simulink model "bidireUnitfinal"  (R2024b)
settings: Solver=VariableStepAuto  StartTime=0.0  StopTime=10  RelTol=1e-3
model workspace (MAT data in the model file):
  charge = 1
undefined symbols (not defined in the file): Ion, Lithium
libraries: spsSeriesRLCBranchLib x3, spsBatteryLib x2, spsMosfetLib x2, spsVoltageMeasurementLib x2, spsCurrentMeasurementLib x1, slpidlib x1, spsTriangleGeneratorLib x1, spspowerguiLib x1
settings Model: Creator=pansi  LastModifiedBy=ASUS

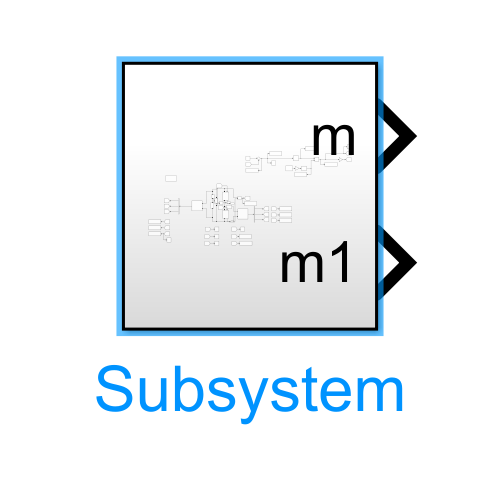
[thumbnail: Simulink's stored preview of the top-level diagram]
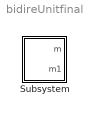
== system bidireUnitfinal ==
  Subsystem : Subsystem

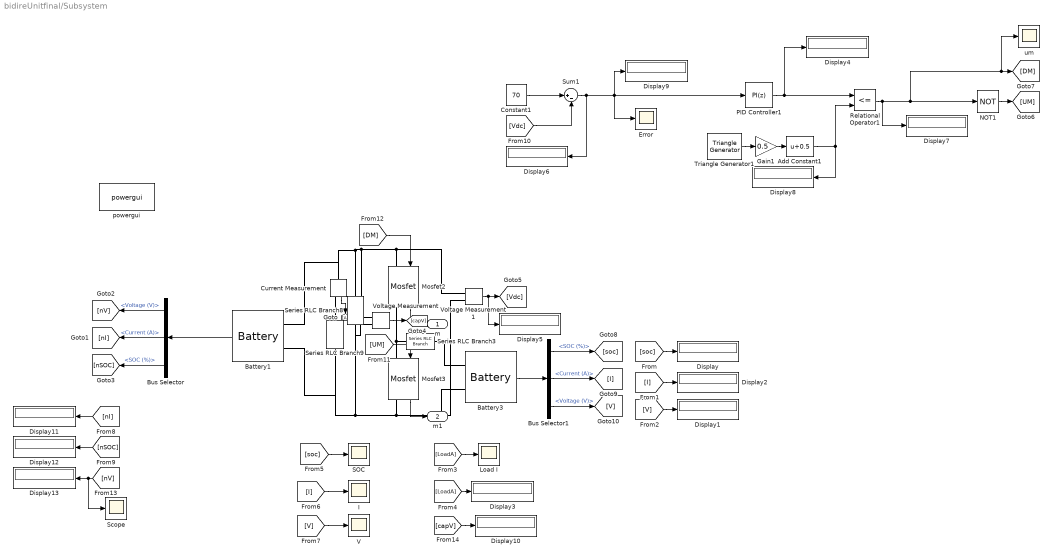
== system bidireUnitfinal/Subsystem ==
  Add Constant1 : Bias  Bias=0.5  SaturateOnIntegerOverflow=off
  Battery1 : spsBatteryLib/Battery  BatType=Lithium-Ion  NomV=25  NomQ=20  SOC=60  Batt_Tr=30  PresetModel=on  MaxQ=20  MinV=18.75  FullV=29.0997  Dis_rate=8.6957  R=0.0125  Normal_OP=18.087  expZone="[27.0096     0.982609]"
  Battery3 : spsBatteryLib/Battery  BatType=Lithium-Ion  NomV=50  NomQ=20  SOC=60  Batt_Tr=30  PresetModel=on  MaxQ=20  MinV=37.5  FullV=58.1994  Dis_rate=8.6957  R=0.025  Normal_OP=18.087  expZone="[54.0193     0.982609]"
  Bus Selector : BusSelector  OutputSignals=Voltage (V),Current (A),SOC (%)
  Bus Selector1 : BusSelector  OutputSignals=SOC (%),Current (A),Voltage (V)
  Constant1 : Constant  Value=70
  Current Measurement : spsCurrentMeasurementLib/Current Measurement  PhasorSimulation=off  OutputType=Complex  PSBequivalent=0
  Display{,1..13} (14 alike) : Display
  Error : Scope
  Gain1 : Gain  Gain=0.5
  Goto : Goto
  I : Scope
  Load I : Scope
  Mosfet2 : spsMosfetLib/Mosfet  Ron=0.1  Lon=0  Rd=0.01  Vfd=0  IC=0  Rs=1e6  Cs=inf  Measurements=on
  Mosfet3 : spsMosfetLib/Mosfet  Ron=0.1  Lon=0  Rd=0.01  Vfd=0  IC=0  Rs=1e6  Cs=inf  Measurements=on
  NOT1 : Logic  Operator=NOT  IconShape=distinctive  AllPortsSameDT=off  OutDataTypeStr=boolean
  PID Controller1 : slpidlib/PID Controller  Controller=PI  Form=Parallel  TimeDomain=Discrete-time  UseExternalTs=off  SampleTime=-1  IntegratorMethod=Forward Euler  FilterMethod=Forward Euler  ControllerParametersSource=internal  P=1  I=50  UseKiTs=off  D=0  UseExternalDerivativeSource=off  N=100  UseFilter=on  TunerSelectOption=Transfer Function Based (PID Tuner App)  ZeroCross=off  InitialConditionSource=internal  InitialConditionForIntegrator=0  InitialConditionForFilter=0  DifferentiatorICPrevScaledInput=0  ExternalReset=none  TrackingMode=off  Kt=1  LimitOutput=on  SatLimitsSource=internal  UpperSaturationLimit=1  LowerSaturationLimit=-1  LinearizeAsGain=on  AntiWindupMode=back-calculation  Kb=1  LimitIntegrator=off  UpperIntegratorSaturationLimit=inf  LowerIntegratorSaturationLimit=-inf  POutMin=[]  POutMax=[]  IOutMin=[]  IOutMax=[]  DOutMin=[]  DOutMax=[]  NOutMin=[]  NOutMax=[]  SumOutMin=[]  SumOutMax=[]  SaturationOutMin=[]  SaturationOutMax=[]  PParamMin=[]  PParamMax=[]  IParamMin=[]  IParamMax=[]  DParamMin=[]  DParamMax=[]  NParamMin=[]  NParamMax=[]  KbParamMin=[]  KbParamMax=[]  KtParamMin=[]  KtParamMax=[]  KbOutMin=[]  KbOutMax=[]  KtOutMin=[]  KtOutMax=[]  IntegratorOutMin=[]  IntegratorOutMax=[]  FilterOutMin=[]  FilterOutMax=[]  SumI1OutMin=[]  SumI1OutMax=[]  SumI2OutMin=[]  SumI2OutMax=[]  SumI3OutMin=[]  SumI3OutMax=[]  SumI4OutMin=[]  SumI4OutMax=[]  SumDOutMin=[]  SumDOutMax=[]  DifferentiatorOutMin=[]  DifferentiatorOutMax=[]  FilterDiffOutCoefMin=[]  FilterDiffOutCoefMax=[]  ReciprocalOutMin=[]  ReciprocalOutMax=[]  SumDenOutMin=[]  SumDenOutMax=[]  SumNumOutMin=[]  SumNumOutMax=[]  DivideOutMin=[]  DivideOutMax=[]  UdiffTsProdOutMin=[]  UdiffTsProdOutMax=[]  NTsProdOutMin=[]  NTsProdOutMax=[]  UintegralTsProdOutMin=[]  UintegralTsProdOutMax=[]  UngainTsProdOutMin=[]  UngainTsProdOutMax=[]  ClampingZeroOutDataTypeStr=Inherit: Inherit via back propagation  ClampingZeroOutMin=[]  ClampingZeroOutMax=[]  FilterDenConstantOutDataTypeStr=Inherit: Inherit via back propagation  FilterDenConstantOutMin=[]  FilterDenConstantOutMax=[]  PCopyOutDataTypeStr=Inherit: Inherit via back propagation  PCopyOutMin=[]  PCopyOutMax=[]  NCopyOutDataTypeStr=Inherit: Inherit via back propagation  NCopyOutMin=[]  NCopyOutMax=[]  IntegratorContinuousStateAttributes=''  IntegratorStateMustResolveToSignalObject=off  IntegratorRTWStateStorageClass=Auto  FilterContinuousStateAttributes=''  FilterStateMustResolveToSignalObject=off  FilterRTWStateStorageClass=Auto  ParallelPVariant=InternalParameters  IdealPVariant=Disabled  IVariant=InternalParameters  DVariant=Disabled  IntegratorVariant=Discrete  SatVariant=Enabled  AWVariant=BackCalculation  PCopyVariant=Disabled  TRVariant=Disabled  FdbkBlocksVariant=Forward  IdealPFdbkVariant=Disabled  SatFdbkVariant=Disabled  DerivativeFilterVariant=Disabled  NVariant=Disabled  NCopyVariant=Disabled_SignalSpec  FilterICVariant=Disabled  IntegratorICVariant=InternalICs  ExternalResetVariant=Disabled  TRSumVariant=Passthrough  SumFdbkVariant=Disabled  SumVariant=Sum_PI  TsampFilterVariant=InternalTs  TsampNgainVariant=Passthrough  TsampIntegralVariant=Disabled_SignalSpec  ExternalSaturationOutDataTypeStr=Inherit: Same as second input  DerivativeSourceVariant=Disabled  PreIntVariant=InternalPreInt
  Relational Operator1 : RelationalOperator  Operator=<=  OutDataTypeStr=boolean  RndMeth=Simplest  InputSameDT=off
  SOC : Scope
  Scope : Scope
  Series RLC Branch3 : spsSeriesRLCBranchLib/Series RLC Branch  LConnTagsString=__new0  RConnTagsString=__new0  BranchType=L  Resistance=1  Inductance=500e-6  SetiL0=off  InitialCurrent=0  Capacitance=1e-6  Setx0=off  InitialVoltage=0  Measurements=None
  Series RLC Branch8 : spsSeriesRLCBranchLib/Series RLC Branch  LConnTagsString=__new0  RConnTagsString=__new0  BranchType=RC  Resistance=1  Inductance=1e-3  SetiL0=off  InitialCurrent=0  Capacitance=1500e-6  Setx0=off  InitialVoltage=0  Measurements=None
  Series RLC Branch9 : spsSeriesRLCBranchLib/Series RLC Branch  LConnTagsString=__new0  RConnTagsString=__new0  BranchType=R  Resistance=5  Inductance=1e-3  SetiL0=off  InitialCurrent=0  Capacitance=1500e-6  Setx0=off  InitialVoltage=0  Measurements=None
  Sum1 : Sum  Inputs=|+-
  Triangle Generator1 : spsTriangleGeneratorLib/Triangle Generator  Freq=10000  Phase=0  Ts=1e-6
  V : Scope
  Voltage Measurement : spsVoltageMeasurementLib/Voltage Measurement  PhasorSimulation=off  OutputType=Complex  PSBequivalent=0
  Voltage Measurement1 : spsVoltageMeasurementLib/Voltage Measurement  PhasorSimulation=off  OutputType=Complex  PSBequivalent=0
  powergui : spspowerguiLib/powergui  Priority=1  SimulationMode=Discrete  SampleTime=1e-6  frequency=60  Iterations=50  frequencyindice=0  Pbase=100e6  ErrMax=1e-4  UnitsV=kV  UnitsW=MW  buscounter=0  FunctionMessages=off  echomessages=off  EnableUseOfTLC=off  CurrentSourceSwitches=off  DisableSnubberDevices=off  DisableRonSwitches=off  DisableVfSwitches=off  DisplayEquations=off  AutomaticDiscreteSolvers=off  SolverType=Tustin/Backward Euler (TBE)  Interpol=off  ExternalGateDelay=off  methode=off  Ts=100  x0status=blocks  SPID=on  SwTol=0  HookPort=off  NonlinearTolerance=1e-4  nMaxIteration=100  ContinueOnMaxIteration=off  RestoreLinks=warning  ResistiveCurrentMeasurement=off  Frange=[0:2:500]  Ylog=off  Xlog=on  ShowGrid=off  save=off  variable=ZData  structure=0  ZoomFFT=off  StartTime=0.0  cycles=1  DisplayStyle=1  fundamental=60  FreqAxis=off  MaxFrequency=1000  frequencyindicesteady=1  RmsSteady=1  display=off
  um : Scope
  m : Outport
  m1 : Outport  Port=2
  wires:
  Voltage Measurement1/1 -> Display5/1, [Vdc]
  [UM] -> Mosfet3/1
  Add Constant1/1 -> Display8/1, Relational Operator1/2
  [V] -> Display1/1
  [capV] -> Display10/1
  [I] -> I/1
  Sum1/1 -> Display9/1, PID Controller1/1, Error/1, Display6/1
  Relational Operator1/1 -> um/1, [DM], NOT1/1, Display7/1
  Bus Selector/3 -> [nSOC]  "<SOC (%)>"
  Bus Selector1/1 -> [soc]  "<SOC (%)>"
  PID Controller1/1 -> Relational Operator1/1, Display4/1
  [nV] -> Scope/1, Display13/1
  Current Measurement/1 -> Goto/1
  Gain1/1 -> Add Constant1/1
  Bus Selector/1 -> [nV]  "<Voltage (V)>"
  [soc] -> SOC/1
  [I] -> Display2/1
  Mosfet3/1 -> m1/1
  Battery3/1 -> Bus Selector1/1
  [DM] -> Mosfet2/1
  Bus Selector1/3 -> [V]  "<Voltage (V)>"
  [nI] -> Display11/1
  [LoadA] -> Load I/1
  [V] -> V/1
  NOT1/1 -> [UM]
  [nSOC] -> Display12/1
  Voltage Measurement/1 -> [capV]
  [Vdc] -> Sum1/2
  [LoadA] -> Display3/1
  Triangle Generator1/1 -> Gain1/1
  Constant1/1 -> Sum1/1
  Battery1/1 -> Bus Selector/1
  Bus Selector/2 -> [nI]  "<Current (A)>"
  Bus Selector1/2 -> [I]  "<Current (A)>"
  [soc] -> Display/1
  Mosfet2/1 -> m/1
  connections:
  Current Measurement/RConn1 -- Series RLC Branch9/LConn1
  Battery3/LConn1 -- Series RLC Branch3/LConn1
  Series RLC Branch8/LConn1 -- Battery1/LConn1 -- Current Measurement/LConn1 -- Voltage Measurement1/LConn1 -- Mosfet2/LConn1 -- Voltage Measurement/LConn1
  Battery3/LConn2 -- Series RLC Branch8/RConn1 -- Voltage Measurement/LConn2 -- Battery1/LConn2 -- Series RLC Branch9/RConn1 -- Mosfet3/RConn1 -- Voltage Measurement1/LConn2
  Mosfet2/RConn1 -- Series RLC Branch3/RConn1 -- Mosfet3/LConn1
